simulink model "ZeroOrderHold"  (Simulink 8.7)
settings: Solver=VariableStepAuto  StartTime=0.0  StopTime=10.0  RelTol=1e-3
values from neighbouring files (symbols this model uses):
  dT = 0.1    [ZeroOrderHold_test.m]    (also in ZeroOrderHoldfunc.m = block.DialogPrm(2).Data)
settings Model: Creator=Chaozhe  LastModifiedBy=Chaozhe
settings DataIOCC: LimitDataPoints=off  SaveFormat=Dataset
settings DebuggingCC: UnderspecifiedInitializationDetection=Simplified  MergeDetectMultiDrivingBlocksExec=error
settings HardwareCC: ProdBitPerPointer=64  ProdLargestAtomicFloat=Float  ProdIntDivRoundTo=Zero  ProdEndianess=LittleEndian  ProdWordSize=64  ProdHWDeviceType=Intel->x86-64 (Windows64)
settings ModelReferenceCC: PropagateSignalLabelsOutOfModel=on
settings ConfigComp: CovModelRefEnable=off

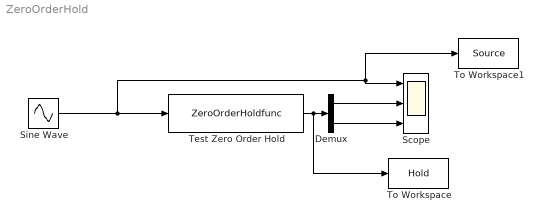
== system ZeroOrderHold ==
  Demux : Demux  Outputs=2
  Scope : Scope  NumInputPorts=3
  Sine Wave : Sin  SampleTime=0
  Test Zero Order Hold : M-S-Function  FunctionName=ZeroOrderHoldfunc  Parameters=0,dT
  To Workspace : ToWorkspace  VariableName=Hold  SaveFormat=Structure With Time  SampleTime=-1
  To Workspace1 : ToWorkspace  VariableName=Source  SaveFormat=Structure With Time  SampleTime=-1
  wires:
  Sine Wave/1 -> To Workspace1/1, Scope/1, Test Zero Order Hold/1
  Test Zero Order Hold/1 -> To Workspace/1, Demux/1
  Demux/1 -> Scope/2
  Demux/2 -> Scope/3
